simulink model "FL1"  (R2018b)
settings: Solver=FixedStepAuto  StartTime=0.0  StopTime=100  FixedStep=0.001  MaxStep=0.001  RelTol=1e-3  EnableMultiTasking=on
InitFcn:
  | A = [0 1; 0 0] ;
  | B = [0 1]' ;
  | K = lqr(A , B , eye(2) , 1 , 0) ;
settings Model: Creator=omid_zandi  LastModifiedBy=Arash
settings OptimizationCC: LifeSpan=inf
settings DebuggingCC: SFUnexpectedBacktrackingDiag=warning  SFNoUnconditionalDefaultTransitionDiag=warning
settings SFSimCC: SimUseLocalCustomCode=off
settings RTWCC: RTWUseLocalCustomCode=off
settings CodeAppCC: StateflowObjectComments=on
settings GRTTargetCC: TargetLangStandard=C89/C90 (ANSI)  GeneratePreprocessorConditionals=Disable all
settings ConfigComp: CovMetricSettings=dw  CovHtmlReporting=on  CovSaveCumulativeToWorkspaceVar=on  CovSaveSingleToWorkspaceVar=on  CovExternalEMLEnable=off

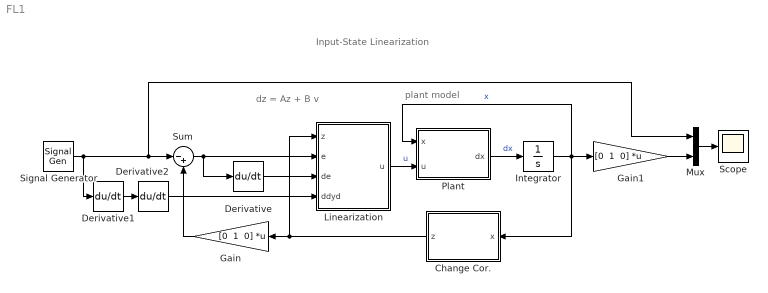
== system FL1 ==
  note: Input-State Linearization
  note: plant model
  note: dz = Az + B v
  Change Cor. : MATLAB Function  TreatAsAtomicUnit=on
  Derivative : Derivative
  Derivative1 : Derivative
  Derivative2 : Derivative
  Gain : Gain  Gain="[0  1  0]"  Multiplication=Matrix(K*u)
  Gain1 : Gain  Gain="[0  1  0]"  Multiplication=Matrix(K*u)
  Integrator : Integrator  InitialCondition=randn(3,1)
  Linearization : MATLAB Function  TreatAsAtomicUnit=on
  Mux : Mux  Inputs=2
  Plant : MATLAB Function  TreatAsAtomicUnit=on
  Scope : Scope
  Signal Generator : SignalGenerator  Frequency=0.05
  Sum : Sum  Inputs=|-+
  wires:
  Integrator/1 -> Gain1/1, Change Cor./1(x), Plant/1(x)  "x"
  Plant/1(dx) -> Integrator/1  "dx"
  Change Cor./1(z) -> Gain/1, Linearization/1(z)
  Signal Generator/1 -> Mux/1, Sum/1, Derivative1/1
  Gain/1 -> Sum/2
  Sum/1 -> Derivative/1, Linearization/2(e)
  Derivative/1 -> Linearization/3(de)
  Derivative1/1 -> Derivative2/1
  Derivative2/1 -> Linearization/4(ddyd)
  Gain1/1 -> Mux/2
  Mux/1 -> Scope/1
  Linearization/1(u) -> Plant/2(u)  "u"

== matlab function FL1/Change Cor. ==
  data: x input; z output
function z = fcn(x)
z = zeros(3, 1);
z(1) = -x(1) + x(3) + atan(x(3)); 
z(2) = x(2);
z(3) = x(3);

== matlab function FL1/Plant ==
  data: x input; u input; dx output
function dx = fcn(x, u)
dx = zeros(3,1); 
dx(1) = -x(1) + (2 + x(3)^2)/(1 + x(3)^2) * u;
dx(2) = x(3) ;
dx(3) = x(1) * x(3) + u ;

== matlab function FL1/Linearization ==
  data: z input; u output; e input; de input; ddyd input
function u = fcn(z, e, de, ddyd)
k1 = 4;
k2 = 4;
v = ddyd - k1 * de - k2 * e;
u = v - z(3) *(-z(1) + z(3) + atan(z(3)));
